simulink model "plant_all_nort"  (Simulink 9.2)
settings: Solver=FixedStepAuto  StartTime=0.0  StopTime=60  FixedStep=1e-3  RelTol=1e-3  EnableMultiTasking=on
undefined symbols (not defined in the file): A, B, C, c, D, g, I, l, m, wn, xi
settings Model: Creator=henrik  LastModifiedBy=henrik
settings DataIOCC: SignalLoggingName=sigsOut
settings OptimizationCC: ExpressionDepthLimit=2147483647  InitFltsAndDblsToZero=on
settings DebuggingCC: SaveWithParameterizedLinksMsg=none  SignalResolutionControl=TryResolveAllWithWarning  MultiTaskDSMMsg=warning  MultiTaskCondExecSysMsg=none
settings HardwareCC: TargetUnknown=on
settings GRTTargetCC: TargetFcnLib=ansi_tfl_tmw.mat  ModelReferenceCompliant=off  MatFileLogging=off

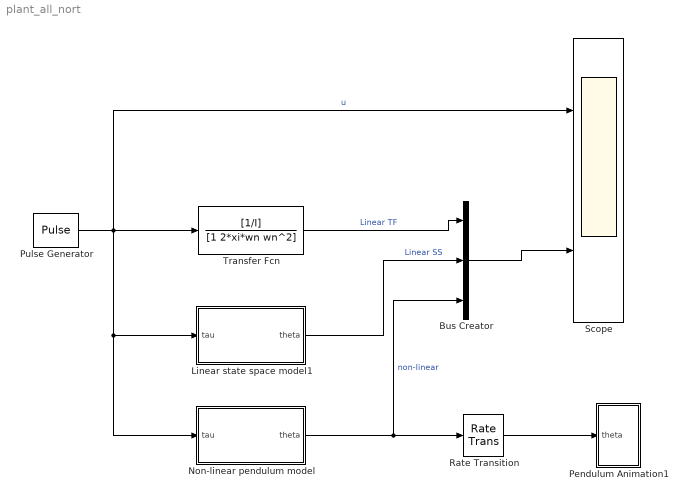
== system plant_all_nort ==
  Bus Creator : BusCreator  Inputs=3
  Linear state space model1 : Subsystem
  Non-linear pendulum model : Subsystem
  Pendulum Animation1 : Subsystem
  Pulse Generator : DiscretePulseGenerator  PulseType=Time based  Period=10  PulseWidth=50  PhaseDelay=1
      settings: AttributesFormatString=Amplitude=%<Amplitude>
  Rate Transition : RateTransition  OutPortSampleTime=0.05
  Scope : Scope  NumInputPorts=2
  Transfer Fcn : TransferFcn  Numerator=[1/I]  Denominator=[1 2*xi*wn wn^2]
  wires:
  Pulse Generator/1 -> Linear state space model1/1(tau), Non-linear pendulum model/1(tau), Scope/1, Transfer Fcn/1  "u"
  Non-linear pendulum model/1(theta) -> Bus Creator/3, Rate Transition/1  "non-linear"
  Bus Creator/1 -> Scope/2
  Transfer Fcn/1 -> Bus Creator/1  "Linear TF"
  Linear state space model1/1(theta) -> Bus Creator/2  "Linear SS"
  Rate Transition/1 -> Pendulum Animation1/1(theta)

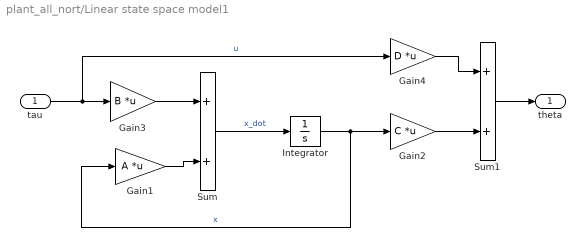
== system plant_all_nort/Linear state space model1 ==
  tau : Inport
  Gain1 : Gain  Gain=A  Multiplication=Matrix(K*u)  SaturateOnIntegerOverflow=on  OutDataTypeStr=Inherit: Same as input  ParamDataTypeStr=Inherit: Same as input
  Gain2 : Gain  Gain=C  Multiplication=Matrix(K*u)  SaturateOnIntegerOverflow=on  OutDataTypeStr=Inherit: Same as input  ParamDataTypeStr=Inherit: Same as input
  Gain3 : Gain  Gain=B  Multiplication=Matrix(K*u)  SaturateOnIntegerOverflow=on  OutDataTypeStr=Inherit: Same as input  ParamDataTypeStr=Inherit: Same as input
  Gain4 : Gain  Gain=D  Multiplication=Matrix(K*u)  SaturateOnIntegerOverflow=on  OutDataTypeStr=Inherit: Same as input  ParamDataTypeStr=Inherit: Same as input
  Integrator : Integrator
  Sum : Sum  SaturateOnIntegerOverflow=on  InputSameDT=on  OutDataTypeStr=Inherit: Same as first input
  Sum1 : Sum  SaturateOnIntegerOverflow=on  InputSameDT=on  OutDataTypeStr=Inherit: Same as first input
  theta : Outport
  wires:
  Sum/1 -> Integrator/1  "x_dot"
  Integrator/1 -> Gain1/1, Gain2/1  "x"
  Gain3/1 -> Sum/1
  tau/1 -> Gain4/1, Gain3/1  "u"
  Gain1/1 -> Sum/2
  Gain2/1 -> Sum1/2
  Gain4/1 -> Sum1/1
  Sum1/1 -> theta/1

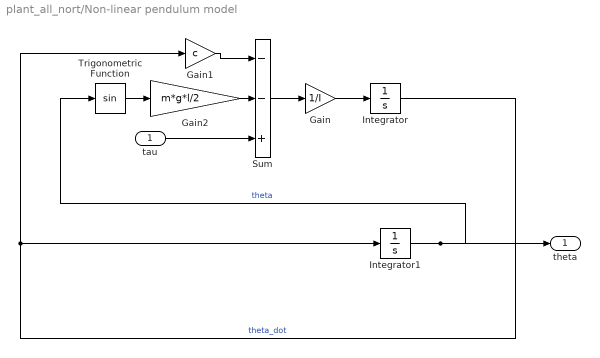
== system plant_all_nort/Non-linear pendulum model ==
  tau : Inport
  Gain : Gain  Gain=1/I  SaturateOnIntegerOverflow=on  OutDataTypeStr=Inherit: Same as input  ParamDataTypeStr=Inherit: Same as input
  Gain1 : Gain  Gain=c  SaturateOnIntegerOverflow=on  OutDataTypeStr=Inherit: Same as input  ParamDataTypeStr=Inherit: Same as input
  Gain2 : Gain  Gain=m*g*l/2  SaturateOnIntegerOverflow=on  OutDataTypeStr=Inherit: Same as input  ParamDataTypeStr=Inherit: Same as input
  Integrator : Integrator
  Integrator1 : Integrator
  Sum : Sum  Inputs=--+  SaturateOnIntegerOverflow=on  InputSameDT=on  OutDataTypeStr=Inherit: Same as first input
  Trigonometric Function : Trigonometry
  theta : Outport
  wires:
  Sum/1 -> Gain/1
  Gain/1 -> Integrator/1
  Gain1/1 -> Sum/1
  Gain2/1 -> Sum/2
  Trigonometric Function/1 -> Gain2/1
  Integrator1/1 -> theta/1, Trigonometric Function/1  "theta"
  Integrator/1 -> Gain1/1, Integrator1/1  "theta_dot"
  tau/1 -> Sum/3

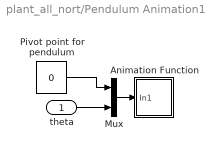
== system plant_all_nort/Pendulum Animation1 ==
  theta : Inport
  Animation Function : Subsystem  mask(Animation Block){ts=0.01}
      mask prompts: ts "Sample time:"
      mask Display: plot([.1,.9],[.9,.9],[.5,.2],[.9,.25],[.475,.475,.525,.525,.475],[.875,.925,.925,.875,.875])
  Mux : Mux  Inputs=2
  Pivot point for pendulum : Constant  Value=0
  wires:
  theta/1 -> Mux/2
  Pivot point for pendulum/1 -> Mux/1
  Mux/1 -> Animation Function/1(In1)

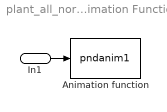
== system plant_all_nort/Pendulum Animation1/Animation Function ==
  In1 : Inport
  Animation function : S-Function  FunctionName=pndanim1  Parameters=ts  SFunctionDeploymentMode=off  EnableBusSupport=off
      settings: DeleteFcn=if ~isempty(findobj('type','figure','name','simppend Animation'));close('simppend Animation'); end;
  wires:
  In1/1 -> Animation function/1
